simulink model "cic_filter_test_newnew_dec5_poly"  (Simulink 7.4)
settings: Solver=ode45  StartTime=0.0  StopTime=10000  RelTol=1e-3
libraries: xbsIndex_r4 x285, simulink x3, xrbsComm_r4 x1, xps_library x1
(part 3 of 3)

== system cic_filter_test_newnew_dec5_poly/npcic_dec5_polyphase1/polynomial4/shift_mult_array ==
  in : Inport
  sync : Inport  Port=2
  adder_tree1 : Subsystem
  adder_tree2 : Subsystem
  delay1 : xbsIndex_r4/Delay  en=off  latency=1  dbl_ovrd=off  reg_retiming=off  block_type=delay
      settings: block_version=11.4
  shift2 : xbsIndex_r4/Shift  shift_dir=Left  shift_bits=1  en=off  latency=0  precision=User Defined  arith_type="Signed  (2's comp)"  n_bits=9  bin_pt=3  quantization=Truncate  overflow=Wrap  dbl_ovrd=off  block_type=shift
  shift5 : xbsIndex_r4/Shift  shift_dir=Left  shift_bits=4  en=off  latency=0  precision=User Defined  arith_type="Signed  (2's comp)"  n_bits=12  bin_pt=3  quantization=Truncate  overflow=Wrap  dbl_ovrd=off  block_type=shift
  sync_delay : xbsIndex_r4/Delay  en=off  latency=2  dbl_ovrd=off  reg_retiming=off  block_type=delay
      settings: block_version=11.4
  out1 : Outport
  out2 : Outport  Port=2
  out3 : Outport  Port=3
  sync_out : Outport  Port=4
  wires:
  in/1 -> adder_tree2/1(sync), adder_tree1/1(sync), shift5/1, shift2/1, adder_tree1/2(din_1), adder_tree2/2(din_1)  "shift_out1"
  shift2/1 -> adder_tree2/3(din_2), adder_tree1/3(din_2)  "shift_out2"
  delay1/1 -> out1/1, out3/1  "out1"
  sync/1 -> sync_delay/1
  adder_tree2/2(dout) -> out2/1  "out2"
  shift5/1 -> adder_tree2/4(din_3)  "shift_out5"
  adder_tree1/2(dout) -> delay1/1  "adder_trees_out1"
  sync_delay/1 -> sync_out/1

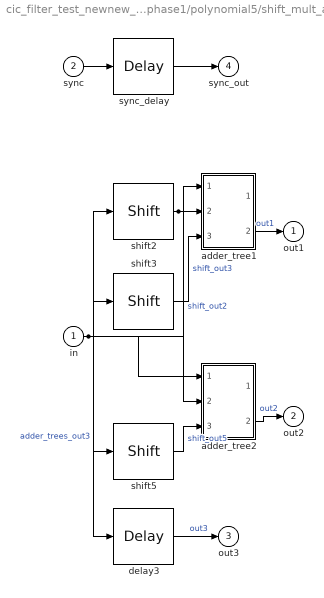
== system cic_filter_test_newnew_dec5_poly/npcic_dec5_polyphase1/polynomial5/shift_mult_array ==
  in : Inport
  sync : Inport  Port=2
  adder_tree1 : Subsystem
  adder_tree2 : Subsystem
  delay3 : xbsIndex_r4/Delay  en=off  latency=1  dbl_ovrd=off  reg_retiming=off  block_type=delay
      settings: block_version=11.4
  shift2 : xbsIndex_r4/Shift  shift_dir=Left  shift_bits=1  en=off  latency=0  precision=User Defined  arith_type="Signed  (2's comp)"  n_bits=9  bin_pt=3  quantization=Truncate  overflow=Wrap  dbl_ovrd=off  block_type=shift
  shift3 : xbsIndex_r4/Shift  shift_dir=Left  shift_bits=2  en=off  latency=0  precision=User Defined  arith_type="Signed  (2's comp)"  n_bits=10  bin_pt=3  quantization=Truncate  overflow=Wrap  dbl_ovrd=off  block_type=shift
  shift5 : xbsIndex_r4/Shift  shift_dir=Left  shift_bits=4  en=off  latency=0  precision=User Defined  arith_type="Signed  (2's comp)"  n_bits=12  bin_pt=3  quantization=Truncate  overflow=Wrap  dbl_ovrd=off  block_type=shift
  sync_delay : xbsIndex_r4/Delay  en=off  latency=1  dbl_ovrd=off  reg_retiming=off  block_type=delay
      settings: block_version=11.4
  out1 : Outport
  out2 : Outport  Port=2
  out3 : Outport  Port=3
  sync_out : Outport  Port=4
  wires:
  in/1 -> shift2/1, shift3/1, shift5/1, adder_tree1/1(sync), adder_tree2/1(sync), delay3/1  "adder_trees_out3"
  shift2/1 -> adder_tree2/2(din_1), adder_tree1/2(din_1)  "shift_out2"
  sync/1 -> sync_delay/1
  adder_tree2/2(dout) -> out2/1  "out2"
  shift3/1 -> adder_tree1/3(din_2)  "shift_out3"
  shift5/1 -> adder_tree2/3(din_2)  "shift_out5"
  adder_tree1/2(dout) -> out1/1  "out1"
  delay3/1 -> out3/1  "out3"
  sync_delay/1 -> sync_out/1

== system cic_filter_test_newnew_dec5_poly/myCIC1/stage1/mult_cxi_blk1/adder_tree2 ==
  sync : Inport
  din_1 : Inport  Port=2
  din_2 : Inport  Port=3
  adder_0 : xbsIndex_r4/AddSub  mode=Addition  use_carryin=off  use_carryout=off  en=off  latency=1  precision=Full  arith_type=Unsigned  n_bits=16  bin_pt=14  quantization="Round  (unbiased: +/- Inf)"  overflow=Saturate  dbl_ovrd=off  use_behavioral_HDL=on  hw_selection=Fabric  pipelined=off  block_type=addsub
  sync_delay : xbsIndex_r4/Delay  en=off  latency=1  dbl_ovrd=off  reg_retiming=off  block_type=delay
      settings: block_version=11.4
  zero_in : xbsIndex_r4/Constant  arith_type=Unsigned  const=0  n_bits=18  bin_pt=17  explicit_period=off  period=1  equ=P=C  opselect=C  inp2=PCIN>>17  opr=+  inp1=P  carry=CIN  dbl_ovrd=off  block_type=constant
      settings: block_version=11.4
  sync_out : Outport
  dout : Outport  Port=2
  wires:
  din_1/1 -> adder_0/2
  sync_delay/1 -> sync_out/1
  sync/1 -> sync_delay/1
  din_2/1 -> adder_0/1
  adder_0/1 -> dout/1

== system cic_filter_test_newnew_dec5_poly/myCIC1/stage1/mult_cxi_blk2/adder_tree1 ==
  sync : Inport
  din_1 : Inport  Port=2
  din_2 : Inport  Port=3
  adder_0 : xbsIndex_r4/AddSub  mode=Addition  use_carryin=off  use_carryout=off  en=off  latency=1  precision=Full  arith_type=Unsigned  n_bits=16  bin_pt=14  quantization="Round  (unbiased: +/- Inf)"  overflow=Saturate  dbl_ovrd=off  use_behavioral_HDL=on  hw_selection=Fabric  pipelined=off  block_type=addsub
  sync_delay : xbsIndex_r4/Delay  en=off  latency=1  dbl_ovrd=off  reg_retiming=off  block_type=delay
      settings: block_version=11.4
  zero_in : xbsIndex_r4/Constant  arith_type=Unsigned  const=0  n_bits=18  bin_pt=17  explicit_period=off  period=1  equ=P=C  opselect=C  inp2=PCIN>>17  opr=+  inp1=P  carry=CIN  dbl_ovrd=off  block_type=constant
      settings: block_version=11.4
  sync_out : Outport
  dout : Outport  Port=2
  wires:
  din_1/1 -> adder_0/2
  sync_delay/1 -> sync_out/1
  sync/1 -> sync_delay/1
  din_2/1 -> adder_0/1
  adder_0/1 -> dout/1

== system cic_filter_test_newnew_dec5_poly/myCIC1/stage1/mult_cxi_blk3/adder_tree2 ==
  sync : Inport
  din_1 : Inport  Port=2
  din_2 : Inport  Port=3
  adder_0 : xbsIndex_r4/AddSub  mode=Addition  use_carryin=off  use_carryout=off  en=off  latency=1  precision=Full  arith_type=Unsigned  n_bits=16  bin_pt=14  quantization="Round  (unbiased: +/- Inf)"  overflow=Saturate  dbl_ovrd=off  use_behavioral_HDL=on  hw_selection=Fabric  pipelined=off  block_type=addsub
  sync_delay : xbsIndex_r4/Delay  en=off  latency=1  dbl_ovrd=off  reg_retiming=off  block_type=delay
      settings: block_version=11.4
  zero_in : xbsIndex_r4/Constant  arith_type=Unsigned  const=0  n_bits=18  bin_pt=17  explicit_period=off  period=1  equ=P=C  opselect=C  inp2=PCIN>>17  opr=+  inp1=P  carry=CIN  dbl_ovrd=off  block_type=constant
      settings: block_version=11.4
  sync_out : Outport
  dout : Outport  Port=2
  wires:
  din_1/1 -> adder_0/2
  sync_delay/1 -> sync_out/1
  sync/1 -> sync_delay/1
  din_2/1 -> adder_0/1
  adder_0/1 -> dout/1

== system cic_filter_test_newnew_dec5_poly/myCIC1/stage1/mult_cxi_blk4/adder_tree1 ==
  sync : Inport
  din_1 : Inport  Port=2
  din_2 : Inport  Port=3
  adder_0 : xbsIndex_r4/AddSub  mode=Addition  use_carryin=off  use_carryout=off  en=off  latency=1  precision=Full  arith_type=Unsigned  n_bits=16  bin_pt=14  quantization="Round  (unbiased: +/- Inf)"  overflow=Saturate  dbl_ovrd=off  use_behavioral_HDL=on  hw_selection=Fabric  pipelined=off  block_type=addsub
  sync_delay : xbsIndex_r4/Delay  en=off  latency=1  dbl_ovrd=off  reg_retiming=off  block_type=delay
      settings: block_version=11.4
  zero_in : xbsIndex_r4/Constant  arith_type=Unsigned  const=0  n_bits=18  bin_pt=17  explicit_period=off  period=1  equ=P=C  opselect=C  inp2=PCIN>>17  opr=+  inp1=P  carry=CIN  dbl_ovrd=off  block_type=constant
      settings: block_version=11.4
  sync_out : Outport
  dout : Outport  Port=2
  wires:
  din_1/1 -> adder_0/2
  sync_delay/1 -> sync_out/1
  sync/1 -> sync_delay/1
  din_2/1 -> adder_0/1
  adder_0/1 -> dout/1

== system cic_filter_test_newnew_dec5_poly/myCIC2/stage1/mult_cxi_blk1/adder_tree2 ==
  sync : Inport
  din_1 : Inport  Port=2
  din_2 : Inport  Port=3
  adder_0 : xbsIndex_r4/AddSub  mode=Addition  use_carryin=off  use_carryout=off  en=off  latency=1  precision=Full  arith_type=Unsigned  n_bits=16  bin_pt=14  quantization="Round  (unbiased: +/- Inf)"  overflow=Saturate  dbl_ovrd=off  use_behavioral_HDL=on  hw_selection=Fabric  pipelined=off  block_type=addsub
  sync_delay : xbsIndex_r4/Delay  en=off  latency=1  dbl_ovrd=off  reg_retiming=off  block_type=delay
      settings: block_version=11.4
  zero_in : xbsIndex_r4/Constant  arith_type=Unsigned  const=0  n_bits=18  bin_pt=17  explicit_period=off  period=1  equ=P=C  opselect=C  inp2=PCIN>>17  opr=+  inp1=P  carry=CIN  dbl_ovrd=off  block_type=constant
      settings: block_version=11.4
  sync_out : Outport
  dout : Outport  Port=2
  wires:
  din_1/1 -> adder_0/2
  sync_delay/1 -> sync_out/1
  sync/1 -> sync_delay/1
  din_2/1 -> adder_0/1
  adder_0/1 -> dout/1

== system cic_filter_test_newnew_dec5_poly/myCIC2/stage1/mult_cxi_blk2/adder_tree1 ==
  sync : Inport
  din_1 : Inport  Port=2
  din_2 : Inport  Port=3
  adder_0 : xbsIndex_r4/AddSub  mode=Addition  use_carryin=off  use_carryout=off  en=off  latency=1  precision=Full  arith_type=Unsigned  n_bits=16  bin_pt=14  quantization="Round  (unbiased: +/- Inf)"  overflow=Saturate  dbl_ovrd=off  use_behavioral_HDL=on  hw_selection=Fabric  pipelined=off  block_type=addsub
  sync_delay : xbsIndex_r4/Delay  en=off  latency=1  dbl_ovrd=off  reg_retiming=off  block_type=delay
      settings: block_version=11.4
  zero_in : xbsIndex_r4/Constant  arith_type=Unsigned  const=0  n_bits=18  bin_pt=17  explicit_period=off  period=1  equ=P=C  opselect=C  inp2=PCIN>>17  opr=+  inp1=P  carry=CIN  dbl_ovrd=off  block_type=constant
      settings: block_version=11.4
  sync_out : Outport
  dout : Outport  Port=2
  wires:
  din_1/1 -> adder_0/2
  sync_delay/1 -> sync_out/1
  sync/1 -> sync_delay/1
  din_2/1 -> adder_0/1
  adder_0/1 -> dout/1

== system cic_filter_test_newnew_dec5_poly/myCIC2/stage1/mult_cxi_blk3/adder_tree2 ==
  sync : Inport
  din_1 : Inport  Port=2
  din_2 : Inport  Port=3
  adder_0 : xbsIndex_r4/AddSub  mode=Addition  use_carryin=off  use_carryout=off  en=off  latency=1  precision=Full  arith_type=Unsigned  n_bits=16  bin_pt=14  quantization="Round  (unbiased: +/- Inf)"  overflow=Saturate  dbl_ovrd=off  use_behavioral_HDL=on  hw_selection=Fabric  pipelined=off  block_type=addsub
  sync_delay : xbsIndex_r4/Delay  en=off  latency=1  dbl_ovrd=off  reg_retiming=off  block_type=delay
      settings: block_version=11.4
  zero_in : xbsIndex_r4/Constant  arith_type=Unsigned  const=0  n_bits=18  bin_pt=17  explicit_period=off  period=1  equ=P=C  opselect=C  inp2=PCIN>>17  opr=+  inp1=P  carry=CIN  dbl_ovrd=off  block_type=constant
      settings: block_version=11.4
  sync_out : Outport
  dout : Outport  Port=2
  wires:
  din_1/1 -> adder_0/2
  sync_delay/1 -> sync_out/1
  sync/1 -> sync_delay/1
  din_2/1 -> adder_0/1
  adder_0/1 -> dout/1

== system cic_filter_test_newnew_dec5_poly/myCIC2/stage1/mult_cxi_blk4/adder_tree1 ==
  sync : Inport
  din_1 : Inport  Port=2
  din_2 : Inport  Port=3
  adder_0 : xbsIndex_r4/AddSub  mode=Addition  use_carryin=off  use_carryout=off  en=off  latency=1  precision=Full  arith_type=Unsigned  n_bits=16  bin_pt=14  quantization="Round  (unbiased: +/- Inf)"  overflow=Saturate  dbl_ovrd=off  use_behavioral_HDL=on  hw_selection=Fabric  pipelined=off  block_type=addsub
  sync_delay : xbsIndex_r4/Delay  en=off  latency=1  dbl_ovrd=off  reg_retiming=off  block_type=delay
      settings: block_version=11.4
  zero_in : xbsIndex_r4/Constant  arith_type=Unsigned  const=0  n_bits=18  bin_pt=17  explicit_period=off  period=1  equ=P=C  opselect=C  inp2=PCIN>>17  opr=+  inp1=P  carry=CIN  dbl_ovrd=off  block_type=constant
      settings: block_version=11.4
  sync_out : Outport
  dout : Outport  Port=2
  wires:
  din_1/1 -> adder_0/2
  sync_delay/1 -> sync_out/1
  sync/1 -> sync_delay/1
  din_2/1 -> adder_0/1
  adder_0/1 -> dout/1

== system cic_filter_test_newnew_dec5_poly/npcic_dec5_polyphase1/polynomial0/shift_mult_array/adder_tree1 ==
  sync : Inport
  din_1 : Inport  Port=2
  din_2 : Inport  Port=3
  adder_0 : xbsIndex_r4/AddSub  mode=Addition  use_carryin=off  use_carryout=off  en=off  latency=1  precision=Full  arith_type=Unsigned  n_bits=16  bin_pt=14  quantization="Round  (unbiased: +/- Inf)"  overflow=Saturate  dbl_ovrd=off  use_behavioral_HDL=on  hw_selection=Fabric  pipelined=off  block_type=addsub
  sync_delay : xbsIndex_r4/Delay  en=off  latency=1  dbl_ovrd=off  reg_retiming=off  block_type=delay
      settings: block_version=11.4
  zero_in : xbsIndex_r4/Constant  arith_type=Unsigned  const=0  n_bits=18  bin_pt=17  explicit_period=off  period=1  equ=P=C  opselect=C  inp2=PCIN>>17  opr=+  inp1=P  carry=CIN  dbl_ovrd=off  block_type=constant
      settings: block_version=11.4
  sync_out : Outport
  dout : Outport  Port=2
  wires:
  din_1/1 -> adder_0/2
  sync_delay/1 -> sync_out/1
  sync/1 -> sync_delay/1
  din_2/1 -> adder_0/1
  adder_0/1 -> dout/1

== system cic_filter_test_newnew_dec5_poly/npcic_dec5_polyphase1/polynomial0/shift_mult_array/adder_tree2 ==
  sync : Inport
  din_1 : Inport  Port=2
  din_2 : Inport  Port=3
  din_3 : Inport  Port=4
  din_4 : Inport  Port=5
  adder_0 : xbsIndex_r4/AddSub  mode=Addition  use_carryin=off  use_carryout=off  en=off  latency=1  precision=Full  arith_type=Unsigned  n_bits=16  bin_pt=14  quantization="Round  (unbiased: +/- Inf)"  overflow=Saturate  dbl_ovrd=off  use_behavioral_HDL=on  hw_selection=Fabric  pipelined=off  block_type=addsub
  adder_1 : xbsIndex_r4/AddSub  mode=Addition  use_carryin=off  use_carryout=off  en=off  latency=1  precision=Full  arith_type=Unsigned  n_bits=16  bin_pt=14  quantization="Round  (unbiased: +/- Inf)"  overflow=Saturate  dbl_ovrd=off  use_behavioral_HDL=on  hw_selection=Fabric  pipelined=off  block_type=addsub
  adder_2 : xbsIndex_r4/AddSub  mode=Addition  use_carryin=off  use_carryout=off  en=off  latency=1  precision=Full  arith_type=Unsigned  n_bits=16  bin_pt=14  quantization="Round  (unbiased: +/- Inf)"  overflow=Saturate  dbl_ovrd=off  use_behavioral_HDL=on  hw_selection=Fabric  pipelined=off  block_type=addsub
  sync_delay : xbsIndex_r4/Delay  en=off  latency=2  dbl_ovrd=off  reg_retiming=off  block_type=delay
      settings: block_version=11.4
  zero_in : xbsIndex_r4/Constant  arith_type=Unsigned  const=0  n_bits=18  bin_pt=17  explicit_period=off  period=1  equ=P=C  opselect=C  inp2=PCIN>>17  opr=+  inp1=P  carry=CIN  dbl_ovrd=off  block_type=constant
      settings: block_version=11.4
  sync_out : Outport
  dout : Outport  Port=2
  wires:
  adder_0/1 -> adder_2/2
  din_4/1 -> adder_1/1
  din_1/1 -> adder_0/2
  sync_delay/1 -> sync_out/1
  sync/1 -> sync_delay/1
  din_2/1 -> adder_0/1
  din_3/1 -> adder_1/2
  adder_1/1 -> adder_2/1
  adder_2/1 -> dout/1

== system cic_filter_test_newnew_dec5_poly/npcic_dec5_polyphase1/polynomial2/shift_mult_array/adder_tree1 ==
  sync : Inport
  din_1 : Inport  Port=2
  din_2 : Inport  Port=3
  din_3 : Inport  Port=4
  din_4 : Inport  Port=5
  adder_0 : xbsIndex_r4/AddSub  mode=Addition  use_carryin=off  use_carryout=off  en=off  latency=1  precision=Full  arith_type=Unsigned  n_bits=16  bin_pt=14  quantization="Round  (unbiased: +/- Inf)"  overflow=Saturate  dbl_ovrd=off  use_behavioral_HDL=on  hw_selection=Fabric  pipelined=off  block_type=addsub
  adder_1 : xbsIndex_r4/AddSub  mode=Addition  use_carryin=off  use_carryout=off  en=off  latency=1  precision=Full  arith_type=Unsigned  n_bits=16  bin_pt=14  quantization="Round  (unbiased: +/- Inf)"  overflow=Saturate  dbl_ovrd=off  use_behavioral_HDL=on  hw_selection=Fabric  pipelined=off  block_type=addsub
  adder_2 : xbsIndex_r4/AddSub  mode=Addition  use_carryin=off  use_carryout=off  en=off  latency=1  precision=Full  arith_type=Unsigned  n_bits=16  bin_pt=14  quantization="Round  (unbiased: +/- Inf)"  overflow=Saturate  dbl_ovrd=off  use_behavioral_HDL=on  hw_selection=Fabric  pipelined=off  block_type=addsub
  sync_delay : xbsIndex_r4/Delay  en=off  latency=2  dbl_ovrd=off  reg_retiming=off  block_type=delay
      settings: block_version=11.4
  zero_in : xbsIndex_r4/Constant  arith_type=Unsigned  const=0  n_bits=18  bin_pt=17  explicit_period=off  period=1  equ=P=C  opselect=C  inp2=PCIN>>17  opr=+  inp1=P  carry=CIN  dbl_ovrd=off  block_type=constant
      settings: block_version=11.4
  sync_out : Outport
  dout : Outport  Port=2
  wires:
  adder_0/1 -> adder_2/2
  din_4/1 -> adder_1/1
  din_1/1 -> adder_0/2
  sync_delay/1 -> sync_out/1
  sync/1 -> sync_delay/1
  din_2/1 -> adder_0/1
  din_3/1 -> adder_1/2
  adder_1/1 -> adder_2/1
  adder_2/1 -> dout/1

== system cic_filter_test_newnew_dec5_poly/npcic_dec5_polyphase1/polynomial2/shift_mult_array/adder_tree2 ==
  sync : Inport
  din_1 : Inport  Port=2
  din_2 : Inport  Port=3
  adder_0 : xbsIndex_r4/AddSub  mode=Addition  use_carryin=off  use_carryout=off  en=off  latency=1  precision=Full  arith_type=Unsigned  n_bits=16  bin_pt=14  quantization="Round  (unbiased: +/- Inf)"  overflow=Saturate  dbl_ovrd=off  use_behavioral_HDL=on  hw_selection=Fabric  pipelined=off  block_type=addsub
  sync_delay : xbsIndex_r4/Delay  en=off  latency=1  dbl_ovrd=off  reg_retiming=off  block_type=delay
      settings: block_version=11.4
  zero_in : xbsIndex_r4/Constant  arith_type=Unsigned  const=0  n_bits=18  bin_pt=17  explicit_period=off  period=1  equ=P=C  opselect=C  inp2=PCIN>>17  opr=+  inp1=P  carry=CIN  dbl_ovrd=off  block_type=constant
      settings: block_version=11.4
  sync_out : Outport
  dout : Outport  Port=2
  wires:
  din_1/1 -> adder_0/2
  sync_delay/1 -> sync_out/1
  sync/1 -> sync_delay/1
  din_2/1 -> adder_0/1
  adder_0/1 -> dout/1

== system cic_filter_test_newnew_dec5_poly/npcic_dec5_polyphase1/polynomial3/shift_mult_array/adder_tree2 ==
  sync : Inport
  din_1 : Inport  Port=2
  din_2 : Inport  Port=3
  adder_0 : xbsIndex_r4/AddSub  mode=Addition  use_carryin=off  use_carryout=off  en=off  latency=1  precision=Full  arith_type=Unsigned  n_bits=16  bin_pt=14  quantization="Round  (unbiased: +/- Inf)"  overflow=Saturate  dbl_ovrd=off  use_behavioral_HDL=on  hw_selection=Fabric  pipelined=off  block_type=addsub
  sync_delay : xbsIndex_r4/Delay  en=off  latency=1  dbl_ovrd=off  reg_retiming=off  block_type=delay
      settings: block_version=11.4
  zero_in : xbsIndex_r4/Constant  arith_type=Unsigned  const=0  n_bits=18  bin_pt=17  explicit_period=off  period=1  equ=P=C  opselect=C  inp2=PCIN>>17  opr=+  inp1=P  carry=CIN  dbl_ovrd=off  block_type=constant
      settings: block_version=11.4
  sync_out : Outport
  dout : Outport  Port=2
  wires:
  din_1/1 -> adder_0/2
  sync_delay/1 -> sync_out/1
  sync/1 -> sync_delay/1
  din_2/1 -> adder_0/1
  adder_0/1 -> dout/1

== system cic_filter_test_newnew_dec5_poly/npcic_dec5_polyphase1/polynomial3/shift_mult_array/adder_tree3 ==
  sync : Inport
  din_1 : Inport  Port=2
  din_2 : Inport  Port=3
  adder_0 : xbsIndex_r4/AddSub  mode=Addition  use_carryin=off  use_carryout=off  en=off  latency=1  precision=Full  arith_type=Unsigned  n_bits=16  bin_pt=14  quantization="Round  (unbiased: +/- Inf)"  overflow=Saturate  dbl_ovrd=off  use_behavioral_HDL=on  hw_selection=Fabric  pipelined=off  block_type=addsub
  sync_delay : xbsIndex_r4/Delay  en=off  latency=1  dbl_ovrd=off  reg_retiming=off  block_type=delay
      settings: block_version=11.4
  zero_in : xbsIndex_r4/Constant  arith_type=Unsigned  const=0  n_bits=18  bin_pt=17  explicit_period=off  period=1  equ=P=C  opselect=C  inp2=PCIN>>17  opr=+  inp1=P  carry=CIN  dbl_ovrd=off  block_type=constant
      settings: block_version=11.4
  sync_out : Outport
  dout : Outport  Port=2
  wires:
  din_1/1 -> adder_0/2
  sync_delay/1 -> sync_out/1
  sync/1 -> sync_delay/1
  din_2/1 -> adder_0/1
  adder_0/1 -> dout/1

== system cic_filter_test_newnew_dec5_poly/npcic_dec5_polyphase1/polynomial4/shift_mult_array/adder_tree1 ==
  sync : Inport
  din_1 : Inport  Port=2
  din_2 : Inport  Port=3
  adder_0 : xbsIndex_r4/AddSub  mode=Addition  use_carryin=off  use_carryout=off  en=off  latency=1  precision=Full  arith_type=Unsigned  n_bits=16  bin_pt=14  quantization="Round  (unbiased: +/- Inf)"  overflow=Saturate  dbl_ovrd=off  use_behavioral_HDL=on  hw_selection=Fabric  pipelined=off  block_type=addsub
  sync_delay : xbsIndex_r4/Delay  en=off  latency=1  dbl_ovrd=off  reg_retiming=off  block_type=delay
      settings: block_version=11.4
  zero_in : xbsIndex_r4/Constant  arith_type=Unsigned  const=0  n_bits=18  bin_pt=17  explicit_period=off  period=1  equ=P=C  opselect=C  inp2=PCIN>>17  opr=+  inp1=P  carry=CIN  dbl_ovrd=off  block_type=constant
      settings: block_version=11.4
  sync_out : Outport
  dout : Outport  Port=2
  wires:
  din_1/1 -> adder_0/2
  sync_delay/1 -> sync_out/1
  sync/1 -> sync_delay/1
  din_2/1 -> adder_0/1
  adder_0/1 -> dout/1

== system cic_filter_test_newnew_dec5_poly/npcic_dec5_polyphase1/polynomial4/shift_mult_array/adder_tree2 ==
  sync : Inport
  din_1 : Inport  Port=2
  din_2 : Inport  Port=3
  din_3 : Inport  Port=4
  adder_0 : xbsIndex_r4/AddSub  mode=Addition  use_carryin=off  use_carryout=off  en=off  latency=1  precision=Full  arith_type=Unsigned  n_bits=16  bin_pt=14  quantization="Round  (unbiased: +/- Inf)"  overflow=Saturate  dbl_ovrd=off  use_behavioral_HDL=on  hw_selection=Fabric  pipelined=off  block_type=addsub
  adder_2 : xbsIndex_r4/AddSub  mode=Addition  use_carryin=off  use_carryout=off  en=off  latency=1  precision=Full  arith_type=Unsigned  n_bits=16  bin_pt=14  quantization="Round  (unbiased: +/- Inf)"  overflow=Saturate  dbl_ovrd=off  use_behavioral_HDL=on  hw_selection=Fabric  pipelined=off  block_type=addsub
  delay_1 : xbsIndex_r4/Delay  en=off  latency=1  dbl_ovrd=off  reg_retiming=off  block_type=delay
      settings: block_version=11.4
  sync_delay : xbsIndex_r4/Delay  en=off  latency=2  dbl_ovrd=off  reg_retiming=off  block_type=delay
      settings: block_version=11.4
  zero_in : xbsIndex_r4/Constant  arith_type=Unsigned  const=0  n_bits=18  bin_pt=17  explicit_period=off  period=1  equ=P=C  opselect=C  inp2=PCIN>>17  opr=+  inp1=P  carry=CIN  dbl_ovrd=off  block_type=constant
      settings: block_version=11.4
  sync_out : Outport
  dout : Outport  Port=2
  wires:
  adder_0/1 -> adder_2/2
  din_2/1 -> adder_0/1
  sync/1 -> sync_delay/1
  sync_delay/1 -> sync_out/1
  din_1/1 -> adder_0/2
  din_3/1 -> delay_1/1
  delay_1/1 -> adder_2/1
  adder_2/1 -> dout/1

== system cic_filter_test_newnew_dec5_poly/npcic_dec5_polyphase1/polynomial5/shift_mult_array/adder_tree1 ==
  sync : Inport
  din_1 : Inport  Port=2
  din_2 : Inport  Port=3
  adder_0 : xbsIndex_r4/AddSub  mode=Addition  use_carryin=off  use_carryout=off  en=off  latency=1  precision=Full  arith_type=Unsigned  n_bits=16  bin_pt=14  quantization="Round  (unbiased: +/- Inf)"  overflow=Saturate  dbl_ovrd=off  use_behavioral_HDL=on  hw_selection=Fabric  pipelined=off  block_type=addsub
  sync_delay : xbsIndex_r4/Delay  en=off  latency=1  dbl_ovrd=off  reg_retiming=off  block_type=delay
      settings: block_version=11.4
  zero_in : xbsIndex_r4/Constant  arith_type=Unsigned  const=0  n_bits=18  bin_pt=17  explicit_period=off  period=1  equ=P=C  opselect=C  inp2=PCIN>>17  opr=+  inp1=P  carry=CIN  dbl_ovrd=off  block_type=constant
      settings: block_version=11.4
  sync_out : Outport
  dout : Outport  Port=2
  wires:
  din_1/1 -> adder_0/2
  sync_delay/1 -> sync_out/1
  sync/1 -> sync_delay/1
  din_2/1 -> adder_0/1
  adder_0/1 -> dout/1

== system cic_filter_test_newnew_dec5_poly/npcic_dec5_polyphase1/polynomial5/shift_mult_array/adder_tree2 ==
  sync : Inport
  din_1 : Inport  Port=2
  din_2 : Inport  Port=3
  adder_0 : xbsIndex_r4/AddSub  mode=Addition  use_carryin=off  use_carryout=off  en=off  latency=1  precision=Full  arith_type=Unsigned  n_bits=16  bin_pt=14  quantization="Round  (unbiased: +/- Inf)"  overflow=Saturate  dbl_ovrd=off  use_behavioral_HDL=on  hw_selection=Fabric  pipelined=off  block_type=addsub
  sync_delay : xbsIndex_r4/Delay  en=off  latency=1  dbl_ovrd=off  reg_retiming=off  block_type=delay
      settings: block_version=11.4
  zero_in : xbsIndex_r4/Constant  arith_type=Unsigned  const=0  n_bits=18  bin_pt=17  explicit_period=off  period=1  equ=P=C  opselect=C  inp2=PCIN>>17  opr=+  inp1=P  carry=CIN  dbl_ovrd=off  block_type=constant
      settings: block_version=11.4
  sync_out : Outport
  dout : Outport  Port=2
  wires:
  din_1/1 -> adder_0/2
  sync_delay/1 -> sync_out/1
  sync/1 -> sync_delay/1
  din_2/1 -> adder_0/1
  adder_0/1 -> dout/1
